simulink model "car_model_FIXED"  (R2022b)
settings: Solver=VariableStepAuto  StartTime=0.0  StopTime=60  RelTol=1e-3
values from neighbouring files (symbols this model uses):
  ABS_MAX_TORQUE = [25 25 25 25]    [Startup.m]
  ABS_MAX_TRQ_CMD = dot(ABS_MAX_TORQUE, MOTOR_ENABLE)    [Startup.m]
  ABS_MIN_TORQUE = [0.01 0.01 0.01 0.01]    [Startup.m]
  acc_IC = 0    [Startup.m]
  ACCELERATION_MAX = 30    [Startup.m]
  ang_IC = 0    [Startup.m]
  ang_vel_IC = 0    [Startup.m]
  ax = Reference_Signals.Chassis_Acceleration_VNED.ax.Data(:)    [Simulation_Data_Parse.m]    (also in Vehicle_Sim_Parse.m)
  ay = Reference_Signals.Chassis_Acceleration_VNED.ay.Data(:)    [Simulation_Data_Parse.m]    (also in Vehicle_Sim_Parse.m)
  az = Reference_Signals.Chassis_Acceleration_VNED.az.Data(:)    [Simulation_Data_Parse.m]    (also in Vehicle_Sim_Parse.m)
  battery_current_IC = 0    [Startup.m]
  BATTERY_CURRENT_MAX = 140    [Startup.m]
  BATTERY_CURRENT_MIN = 0    [Startup.m]
  battery_FT_IC = 300    [Startup.m]
  battery_T_IC = 300    [Startup.m]
  BATTERY_TEMPERATURE_MAX = 60    [Startup.m]
  BATTERY_TEMPERATURE_MIN = 0    [Startup.m]
  battery_voltage_IC = Ns*max(Em)    [Startup.m]
  BATTERY_VOLTAGE_MAX = 340    [Startup.m]
  BATTERY_VOLTAGE_MIN = 60    [Startup.m]
  Brake_Pressure_IC = 1    [Startup.m]
  ccl_IC = 0    [Startup.m]
  CENTER_STEER_ANGLE_MAX = 130    [Startup.m]
  covarience_matrix_IC = Simulink.Parameter(eye(28)./1000)    [Startup.m]
  dcl_IC = 140    [Startup.m]
  DCL_MAX = 130    [Startup.m]
  DCL_MIN = 0    [Startup.m]
  driver_t = 0.015    [Startup.m]
  fusion_t = Simulink.Parameter(0.01)    [Startup.m]
  fusion_t_sim = fusion_t.copy    [Startup.m]
  Fz_IC = m_all*g/4    [Startup.m]
  g = 9.81    [Startup.m]
  gps_hz = 0.01    [Startup.m]
  gps_ratio = Simulink.Parameter(gps_hz / imu_hz.Value)    [Startup.m]
  imu_hz = fusion_t.copy    [Startup.m]
  location_lla_IC = Simulink.Parameter([40.437675, -86.943750, 200])    [Startup.m]
  MAG_MAX = 200    [Startup.m]
  Max_Brake_Pressure = 10^8    (= 100000000)    [Startup.m]
  Max_Driver_Input = 1    [Startup.m]
  MAX_DTHETA_DRIVER = 360    [Startup.m]
  MAX_STEERING_ADJUST = 15    [Startup.m]
  Min_Brake_Pressure = 1    [Startup.m]
  Min_Driver_Input = 0    [Startup.m]
  motor_current_IC = 0    [Startup.m]
  MOTOR_CURRENT_MAX = 70    [Startup.m]
  MOTOR_CURRENT_MIN = 0    [Startup.m]
  MOTOR_ENABLE = [0 0 1 1]    [Startup.m]
  motor_FT_IC = 300    [Startup.m]
  motor_T_IC = 300    [Startup.m]
  MOTOR_TEMPERATURE_MAX = 100    [Startup.m]
  MOTOR_TEMPERATURE_MIN = 0    [Startup.m]
  motor_voltage_IC = 332    [Startup.m]
  MOTOR_VOLTAGE_MAX = 340    [Startup.m]
  MOTOR_VOLTAGE_MIN = 90    [Startup.m]
  omega_IC = 0    [Startup.m]
  OMEGA_MAX = 150    [Startup.m]
  OMEGA_MIN = 0    [Startup.m]
  ORIENTATION_MAX = 360    [Startup.m]
  pos_IC = 0    [Startup.m]
  POS_MAX = 300    [Startup.m]
  rho = 1.225    [Startup.m]
  selected_maxvm = MIN_TRACK_DATA.(event_names(10))    [Startup.m]
  selected_sweep = ALL_SWEEP_DATA.(sweep_names(1))    [Startup.m]
  selected_track = ALL_TRACK_DATA.(event_names(10))    [Startup.m]
  shock_length_IC = 0.1    [Startup.m]
  SHOCK_LENGTH_MAX = 0.25    [Startup.m]
  SHOCK_LENGTH_MIN = 0    [Startup.m]
  state_IC = zeros(28,1)    [Startup.m]
  theta_IC = 0    [Startup.m]
  TRACTION_ENABLE = 0    [Startup.m]
  TVS_ENABLE = 0    [Startup.m]
  tvs_t = 0.015    [Startup.m]
  tvs_t_sim = tvs_t    (= 0.015)    [Startup.m]
  Tx_I = 0    [Startup.m]
  vel_IC = [0 0 0]    [Startup.m]
  VELOCITY_MAX = 30    [Startup.m]
  X = Reference_Signals.Chassis_Position.X.Data(:)    [Simulation_Data_Parse.m]    (also in Vehicle_Sim_Parse.m = Chassis_Signals.InertFrm.Cg.Disp.X.Data(:))
  Y = Reference_Signals.Chassis_Position.Y.Data(:)    [Simulation_Data_Parse.m]    (also in Vehicle_Sim_Parse.m = Chassis_Signals.InertFrm.Cg.Disp.Y.Data(:))
  YAW_ENABLE = 1    [Startup.m]
  YAW_MAX = 2.5    [Startup.m]
undefined symbols (not defined in the file or in its folder): ActSuspDutyCycle, Aeq_left, Aeq_right, alpha_error, ang_acc_hystersesis, area_air, axb, br, brake_bias, covA, covG, covM, covP, covV, CURRENT_BUFFER, cy_sweep, dB, deadband_angle, dIndex, DiscIntNeverNeededParam, dt_OFF, dt_ON, dTx, dx, dZ, efficiency_grid, F0z, forward_look_straight, forward_look_turn, Fz_sweep, GAIN_ABS, gearbox_efficiency, gr, I, I_Driver, IMU_accel, IMU_gyro, IMU_mag, IMUNED2VNED, indicies, IYY, kx_sweep, l, lambda_star, low_V_SA, lr, m_all, m_body, m_unsprung, MAGNED2VNED, MAX_I_Driver, max_yaw, min_velocity_regen, motorControllerCurve, motorTempCurve, motorTempX, mu_star, mx_sweep, my_sweep, noise_state ... (+40)
libraries: fl_lib x82, nesl_utility x32, vehdynlibtire x10, vehdynlibsuspension x8, simulink x5, autolibutils x5, sharedtransform x5, sdl_lib x4, EngineCoolingComponents_lib x4, slpidlib x3, SimscapeFluids_lib x3, shared6dof x2
(part 2 of 14)

== system car_model_FIXED/Driver & Environment/Reference Generator ==
  Analog Signals : Inport
  Driver Information : BusCreator  Inputs=12
  Memory : Memory  InitialCondition=1
  Memory1 : Memory  InitialCondition=1
  Reference Geneator : MATLAB Function  TreatAsAtomicUnit=on  SystemSampleTime=driver_t
  Selector : BusSelector  OutputSignals=psi,Vel,r,Disp,Omega
  Subsystem : Subsystem
  To Workspace : ToWorkspace  VariableName=Driver_Signals  SaveFormat=Timeseries  SampleTime=-1
  Unit Delay : UnitDelay  SampleTime=-1  HasFrameUpgradeWarning=on
  Unit Delay1 : UnitDelay  InitialCondition=1000  SampleTime=-1  HasFrameUpgradeWarning=on
  Controller Information : Outport
  wires:
  Analog Signals/1 -> To Workspace/1, Selector/1  "Driver"
  Selector/1 -> Subsystem/1(<psi>)  "<psi>"
  Reference Geneator/4(d_error) -> Driver Information/2
  Driver Information/1 -> Controller Information/1  "Driver Information"
  Selector/2 -> Reference Geneator/4(Vg)  "<Vel>"
  Reference Geneator/3(v_error) -> Driver Information/1
  Reference Geneator/6(v_cog) -> Driver Information/4
  Subsystem/1(psi_rev) -> Reference Geneator/3(psi)
  Reference Geneator/5(psi_error) -> Driver Information/3
  Reference Geneator/2(index_all) -> Memory/1
  Memory/1 -> Reference Geneator/2("index_all ")
  Reference Geneator/7(r_ref) -> Driver Information/5
  Reference Geneator/8(r_error) -> Driver Information/6
  Reference Geneator/15(ahead) -> Unit Delay/1
  Unit Delay/1 -> Reference Geneator/8("ahead ")
  Reference Geneator/12(omega) -> Driver Information/10
  Reference Geneator/9(x_ref) -> Driver Information/7
  Reference Geneator/10(y_ref) -> Driver Information/8
  Selector/3 -> Reference Geneator/5(yaw)  "<r>"
  Selector/4 -> Reference Geneator/6(pos)  "<Disp>"
  Reference Geneator/11(yaw_ref) -> Driver Information/9
  Memory1/1 -> Reference Geneator/1("index_small ")
  Reference Geneator/1(index_small) -> Memory1/1
  Reference Geneator/16(di_now) -> Unit Delay1/1
  Unit Delay1/1 -> Reference Geneator/9(di_prev)
  Selector/5 -> Reference Geneator/7("omega ")  "<Omega>"
  Reference Geneator/13(p_error) -> Driver Information/11
  Reference Geneator/14(Vnow) -> Driver Information/12

== system car_model_FIXED/Driver & Environment/Sweep Generator ==
  Analog Signals : Inport
  Bus Creator : BusCreator  Inputs=2
  Bus Selector : BusSelector  OutputSignals=Vel
  Memory : Memory  InitialCondition=1
  Sweep Generator : MATLAB Function  TreatAsAtomicUnit=on  SystemSampleTime=driver_t
  To Workspace : ToWorkspace  VariableName=counter  SaveFormat=Timeseries  SampleTime=-1
  Unit Delay : UnitDelay  SampleTime=-1  HasFrameUpgradeWarning=on
  Unit Delay1 : UnitDelay  InitialCondition=1  SampleTime=-1  HasFrameUpgradeWarning=on
  Controller Information : Outport
  wires:
  Analog Signals/1 -> Bus Selector/1
  Sweep Generator/2(vel_err) -> Bus Creator/1  "Velocity Error"
  Sweep Generator/3(ref_steer) -> Bus Creator/2  "Steering Angle"
  Bus Creator/1 -> Controller Information/1
  Bus Selector/1 -> Sweep Generator/2(vel)  "<Vel>"
  Sweep Generator/1(index) -> Memory/1
  Memory/1 -> Sweep Generator/1("index ")
  Sweep Generator/5(counter) -> Unit Delay/1, To Workspace/1
  Unit Delay/1 -> Sweep Generator/4("counter ")
  Sweep Generator/4(ON) -> Unit Delay1/1
  Unit Delay1/1 -> Sweep Generator/3("ON ")

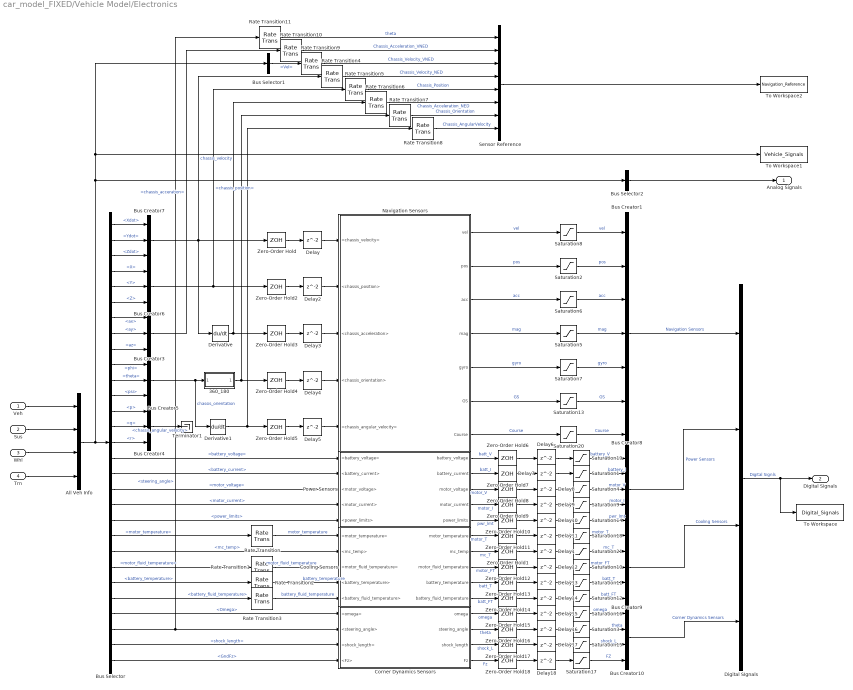
== system car_model_FIXED/Vehicle Model/Electronics ==
  Veh : Inport
  Sus : Inport  Port=2
  Whl : Inport  Port=3
  Trn : Inport  Port=4
  360_180 : Subsystem
  All Veh Info : BusCreator  Inputs=veh,sus,whl,trn
  Bus Creator1 : BusCreator  Inputs=7
  Bus Creator10 : BusCreator  Inputs=4
  Bus Creator3 : BusCreator  Inputs=ax,ay,az
  Bus Creator4 : BusCreator  Inputs=p,q,r
  Bus Creator5 : BusCreator  Inputs=phi,theta,psi
  Bus Creator6 : BusCreator  Inputs=X,Y,Z
  Bus Creator7 : BusCreator  Inputs=Xdot,Ydot,Zdot
  Bus Creator8 : BusCreator  Inputs=5
  Bus Creator9 : BusCreator  Inputs=5
  Bus Selector : BusSelector  OutputSignals=veh.InertFrm.Cg.Vel.Xdot,veh.InertFrm.Cg.Vel.Ydot,veh.InertFrm.Cg.Vel.Zdot,veh.InertFrm.Cg.Disp.X,veh.InertFrm.Cg.Disp.Y,veh.InertFrm.Cg.Disp.Z,veh.BdyFrm.Cg.Acc.ax,veh.BdyFrm.Cg.Acc.ay,veh.BdyFrm.Cg.Acc.az,veh.InertFrm.Cg.Ang.phi,veh.InertFrm.Cg.Ang.theta,veh.InertFrm.Cg.Ang.psi,veh.BdyFrm.Cg.AngVel.p,veh.BdyFrm.Cg.AngVel.q,veh.BdyFrm.Cg.AngVel.r,trn.battery_voltage,trn.battery_current,trn.motor_voltage,trn.motor_current,trn.power_limits,trn.motor_temperature,trn.mc_temp,trn.motor_fluid_temperature,trn.battery_temperature,trn.battery_fluid_temperature,whl.TireFrame.Omega,sus.Sus.steering_angle,sus.Sus.shock_length,whl.TireFrame.GndFz
  Bus Selector1 : BusSelector  OutputSignals=veh.BdyFrm.Cg.Vel
  Bus Selector2 : BusSelector  OutputSignals=veh.InertFrm.Cg.Disp,veh.InertFrm.Cg.Ang.psi,veh.BdyFrm.Cg.Vel,veh.BdyFrm.Cg.AngVel.r,sus.Sus.steering_angle,whl.TireFrame.Omega  OutputAsBus=on
  Cooling Sensors : Subsystem
  Corner Dynamics Sensors : Subsystem
  Delay : Delay  InitialCondition=([1;1]*vel_IC)'
  Delay1 : Delay  InitialCondition=[1 1; 1 1; 1 1; 1 1].*motor_T_IC
  Delay10 : Delay  InitialCondition=[dcl_IC; ccl_IC]*[1 1]
  Delay11 : Delay  InitialCondition=[1 1; 1 1; 1 1; 1 1].*motor_T_IC
  Delay12 : Delay  InitialCondition=[1 1; 1 1].*motor_FT_IC
  Delay13 : Delay  InitialCondition=[1 1].*battery_T_IC
  Delay14 : Delay  InitialCondition=[1 1].*battery_FT_IC
  Delay15 : Delay  InitialCondition=ones(1, 4, 2).*omega_IC
  Delay16 : Delay  InitialCondition=[1 1].*theta_IC
  Delay17 : Delay  InitialCondition=[1 1; 1 1; 1 1; 1 1].*shock_length_IC
  Delay18 : Delay  InitialCondition=[1 1; 1 1; 1 1; 1 1].*Fz_IC
  Delay2 : Delay  InitialCondition=[1 1; 1 1; 1 1].*pos_IC
  Delay3 : Delay  InitialCondition=[1 1; 1 1; 1 1].*acc_IC
  Delay4 : Delay  InitialCondition=[1 1; 1 1; 1 1].*ang_IC
  Delay5 : Delay  InitialCondition=[1 1; 1 1; 1 1].*ang_vel_IC
  Delay6 : Delay  InitialCondition=[1 1].*battery_voltage_IC
  Delay7 : Delay  InitialCondition=[1 1].*battery_current_IC
  Delay8 : Delay  InitialCondition=[1 1; 1 1; 1 1; 1 1].*motor_voltage_IC
  Delay9 : Delay  InitialCondition=ones(1, 4, 2).*motor_current_IC
  Derivative : Derivative
  Derivative1 : Derivative
  Digital SIgnals : BusCreator  Inputs=4
  Navigation Sensors : Subsystem
  Power Sensors : Subsystem
  Rate Transition : RateTransition  OutPortSampleTime=0
  Rate Transition1 : RateTransition  InitialCondition=[1 1].*motor_FT_IC  OutPortSampleTime=0
  Rate Transition{4..11} (8 alike) : RateTransition  Deterministic=off  OutPortSampleTime=fusion_t
  Rate Transition2 : RateTransition  OutPortSampleTime=0
  Rate Transition3 : RateTransition  OutPortSampleTime=0
  Saturation1 : Saturate  UpperLimit=BATTERY_CURRENT_MAX  LowerLimit=BATTERY_CURRENT_MIN
  Saturation10 : Saturate  UpperLimit=MOTOR_TEMPERATURE_MAX  LowerLimit=MOTOR_TEMPERATURE_MIN
  Saturation11 : Saturate  UpperLimit=BATTERY_TEMPERATURE_MAX  LowerLimit=BATTERY_TEMPERATURE_MIN
  Saturation12 : Saturate  UpperLimit=BATTERY_TEMPERATURE_MAX  LowerLimit=BATTERY_TEMPERATURE_MIN
  Saturation13 : Saturate  UpperLimit=VELOCITY_MAX  LowerLimit=-VELOCITY_MAX
  Saturation14 : Saturate  UpperLimit=DCL_MAX  LowerLimit=DCL_MIN
  Saturation15 : Saturate  UpperLimit=SHOCK_LENGTH_MAX  LowerLimit=SHOCK_LENGTH_MIN
  Saturation16 : Saturate  UpperLimit=OMEGA_MAX  LowerLimit=OMEGA_MIN
  Saturation17 : Saturate  UpperLimit=1200  LowerLimit=200
  Saturation18 : Saturate  UpperLimit=MOTOR_TEMPERATURE_MAX  LowerLimit=MOTOR_TEMPERATURE_MIN
  Saturation19 : Saturate  UpperLimit=BATTERY_VOLTAGE_MAX  LowerLimit=BATTERY_VOLTAGE_MIN
  Saturation2 : Saturate  UpperLimit=inf  LowerLimit=-inf
  Saturation20 : Saturate  UpperLimit=ORIENTATION_MAX  LowerLimit=-ORIENTATION_MAX
  Saturation21 : Saturate  UpperLimit=MOTOR_TEMPERATURE_MAX  LowerLimit=MOTOR_TEMPERATURE_MIN
  Saturation3 : Saturate  UpperLimit=CENTER_STEER_ANGLE_MAX  LowerLimit=-CENTER_STEER_ANGLE_MAX
  Saturation4 : Saturate  UpperLimit=MOTOR_VOLTAGE_MAX  LowerLimit=MOTOR_VOLTAGE_MIN
  Saturation5 : Saturate  UpperLimit=MAG_MAX  LowerLimit=-MAG_MAX
  Saturation6 : Saturate  UpperLimit=ACCELERATION_MAX  LowerLimit=-ACCELERATION_MAX
  Saturation7 : Saturate  UpperLimit=YAW_MAX  LowerLimit=-YAW_MAX
  Saturation8 : Saturate  UpperLimit=VELOCITY_MAX  LowerLimit=-VELOCITY_MAX
  Saturation9 : Saturate  UpperLimit=MOTOR_CURRENT_MAX  LowerLimit=MOTOR_CURRENT_MIN
  Sensor Reference : BusCreator  Inputs=8
  Terminator1 : Terminator
  To Workspace : ToWorkspace  VariableName=Digital_Signals  SaveFormat=Timeseries  SampleTime=-1
  To Workspace1 : ToWorkspace  VariableName=Vehicle_Signals  SaveFormat=Timeseries  SampleTime=-1
  To Workspace2 : ToWorkspace  VariableName=Navigation_Reference  SaveFormat=Timeseries  SampleTime=-1
  Zero-Order Hold : ZeroOrderHold  SampleTime=gps_hz
  Zero-Order Hold{1,6..18} (14 alike) : ZeroOrderHold  SampleTime=tvs_t_sim
  Zero-Order Hold2 : ZeroOrderHold  SampleTime=gps_hz
  Zero-Order Hold3 : ZeroOrderHold  SampleTime=imu_hz
  Zero-Order Hold4 : ZeroOrderHold  SampleTime=imu_hz
  Zero-Order Hold5 : ZeroOrderHold  SampleTime=imu_hz
  Analog Signals : Outport
  Digital Signals : Outport  Port=2
  wires:
  Sus/1 -> All Veh Info/2
  Whl/1 -> All Veh Info/3
  Veh/1 -> All Veh Info/1
  Trn/1 -> All Veh Info/4
  Bus Selector/7 -> Bus Creator3/1  "<ax>"
  Bus Selector/8 -> Bus Creator3/2  "<ay>"
  Bus Selector/9 -> Bus Creator3/3  "<az>"
  Bus Selector/13 -> Bus Creator4/1  "<p>"
  Bus Selector/14 -> Bus Creator4/2  "<q>"
  Bus Selector/15 -> Bus Creator4/3  "<r>"
  Bus Selector/1 -> Bus Creator7/1  "<Xdot>"
  Bus Selector/2 -> Bus Creator7/2  "<Ydot>"
  Bus Selector/10 -> Bus Creator5/1  "<phi>"
  Bus Selector/11 -> Bus Creator5/2  "<theta>"
  Bus Selector/12 -> Bus Creator5/3  "<psi>"
  Bus Selector/4 -> Bus Creator6/1  "<X>"
  Bus Selector/5 -> Bus Creator6/2  "<Y>"
  Bus Selector2/1 -> Analog Signals/1
  Bus Selector/3 -> Bus Creator7/3  "<Zdot>"
  Bus Selector/6 -> Bus Creator6/3  "<Z>"
  Bus Creator7/1 -> Zero-Order Hold/1, Rate Transition4/1, Derivative/1  "chassis_velocity"
  Bus Creator6/1 -> Zero-Order Hold2/1, Rate Transition5/1  "<chassis_position>"
  Bus Creator5/1 -> Derivative1/1, 360_180/1(<psi>)  "chassis_orientation"
  Bus Selector/20 -> Power Sensors/5(<power_limits>)  "<power_limits>"
  Bus Selector/17 -> Power Sensors/2(<battery_current>)  "<battery_current>"
  Bus Selector/19 -> Power Sensors/4(<motor_current>)  "<motor_current>"
  Bus Selector/18 -> Power Sensors/3(<motor_voltage>)  "<motor_voltage>"
  Bus Selector/21 -> Rate Transition/1  "<motor_temperature>"
  Bus Selector/26 -> Corner Dynamics Sensors/1(<omega>)  "<Omega>"
  Bus Selector/27 -> Corner Dynamics Sensors/2(<steering_angle>), Rate Transition11/1  "<steering_angle>"
  Bus Selector/28 -> Corner Dynamics Sensors/3(<shock_length>)  "<shock_length>"
  Bus Selector/29 -> Corner Dynamics Sensors/4(<Fz>)  "<GndFz>"
  Bus Selector/23 -> Rate Transition1/1  "<motor_fluid_temperature>"
  Bus Selector/16 -> Power Sensors/1(<battery_voltage>)  "<battery_voltage>"
  Bus Selector/24 -> Rate Transition2/1  "<battery_temperature>"
  Bus Selector/25 -> Rate Transition3/1  "<battery_fluid_temperature>"
  Navigation Sensors/1(vel) -> Saturation8/1  "vel"
  Navigation Sensors/2(pos) -> Saturation2/1  "pos"
  Navigation Sensors/3(acc) -> Saturation6/1  "acc"
  Navigation Sensors/4(mag) -> Saturation5/1  "mag"
  Navigation Sensors/5(gyro) -> Saturation7/1  "gyro"
  Power Sensors/1(battery_voltage) -> Zero-Order Hold6/1  "batt_V"
  Power Sensors/2(battery_current) -> Zero-Order Hold7/1  "batt_I"
  Power Sensors/3(motor_voltage) -> Zero-Order Hold8/1  "motor_V"
  Power Sensors/4(motor_current) -> Zero-Order Hold9/1  "motor_I"
  Power Sensors/5(power_limits) -> Zero-Order Hold10/1  "pwr_lmt"
  Cooling Sensors/1(motor_temperature) -> Zero-Order Hold11/1  "motor_T"
  Cooling Sensors/3(motor_fluid_temperature) -> Zero-Order Hold12/1  "motor_FT"
  Cooling Sensors/4(battery_temperature) -> Zero-Order Hold13/1  "batt_T"
  Cooling Sensors/5(battery_fluid_temperature) -> Zero-Order Hold14/1  "batt_FT"
  Corner Dynamics Sensors/1(omega) -> Zero-Order Hold15/1  "omega"
  Corner Dynamics Sensors/2(steering_angle) -> Zero-Order Hold16/1  "theta"
  Corner Dynamics Sensors/3(shock_length) -> Zero-Order Hold17/1  "shock_L"
  Corner Dynamics Sensors/4(Fz) -> Zero-Order Hold18/1  "Fz"
  Bus Creator1/1 -> Digital SIgnals/1  "Navigation Sensors"
  Bus Creator8/1 -> Digital SIgnals/2  "Power Sensors"
  Bus Creator10/1 -> Digital SIgnals/4  "Corner Dynamics Sensors"
  Digital SIgnals/1 -> Digital Signals/1, To Workspace/1  "Digital Signls"
  Saturation15/1 -> Bus Creator10/3  "shock_L"
  Saturation17/1 -> Bus Creator10/4  "FZ"
  Saturation3/1 -> Bus Creator10/2  "theta"
  Saturation16/1 -> Bus Creator10/1  "omega"
  Saturation8/1 -> Bus Creator1/1  "vel"
  Saturation2/1 -> Bus Creator1/2  "pos"
  Saturation6/1 -> Bus Creator1/3  "acc"
  Saturation5/1 -> Bus Creator1/4  "mag"
  Saturation7/1 -> Bus Creator1/5  "gyro"
  Saturation19/1 -> Bus Creator8/1  "battery_V"
  Saturation1/1 -> Bus Creator8/2  "battery_I"
  Saturation9/1 -> Bus Creator8/4  "motor_I"
  Saturation4/1 -> Bus Creator8/3  "motor_V"
  Saturation14/1 -> Bus Creator8/5  "pwr_lmt"
  Saturation18/1 -> Bus Creator9/1  "motor_T"
  Saturation10/1 -> Bus Creator9/3  "motor_FT"
  Saturation11/1 -> Bus Creator9/4  "batt_T"
  Saturation12/1 -> Bus Creator9/5  "batt_FT"
  Zero-Order Hold6/1 -> Delay6/1
  Zero-Order Hold7/1 -> Delay7/1
  Zero-Order Hold8/1 -> Delay8/1
  Zero-Order Hold9/1 -> Delay9/1
  Zero-Order Hold10/1 -> Delay10/1
  Zero-Order Hold11/1 -> Delay11/1
  Zero-Order Hold12/1 -> Delay12/1
  Zero-Order Hold13/1 -> Delay13/1
  Zero-Order Hold14/1 -> Delay14/1
  Zero-Order Hold15/1 -> Delay15/1
  Zero-Order Hold16/1 -> Delay16/1
  Zero-Order Hold17/1 -> Delay17/1
  Zero-Order Hold18/1 -> Delay18/1
  Delay6/1 -> Saturation19/1
  Delay7/1 -> Saturation1/1
  Delay8/1 -> Saturation4/1
  Delay9/1 -> Saturation9/1
  Delay10/1 -> Saturation14/1
  Delay11/1 -> Saturation18/1
  Delay12/1 -> Saturation10/1
  Delay13/1 -> Saturation11/1
  Delay14/1 -> Saturation12/1
  Delay15/1 -> Saturation16/1
  Delay16/1 -> Saturation3/1
  Delay17/1 -> Saturation15/1
  Delay18/1 -> Saturation17/1
  Rate Transition/1 -> Cooling Sensors/1(<motor_temperature>)  "motor_temperature"
  Rate Transition1/1 -> Cooling Sensors/3(<motor_fluid_temperature>)  "motor_fluid_temperature"
  Rate Transition2/1 -> Cooling Sensors/4(<battery_temperature>)  "battery_temperature"
  Rate Transition3/1 -> Cooling Sensors/5(<battery_fluid_temperature>)  "battery_fluid_temperature"
  Bus Creator9/1 -> Digital SIgnals/3  "Cooling Sensors"
  Navigation Sensors/6(GS) -> Saturation13/1  "GS"
  Navigation Sensors/7(Course) -> Saturation20/1  "Course"
  Saturation13/1 -> Bus Creator1/6  "GS"
  Saturation20/1 -> Bus Creator1/7  "Course"
  Delay/1 -> Navigation Sensors/1(<chassis_velocity>)
  Delay2/1 -> Navigation Sensors/2(<chassis_position>)
  Derivative/1 -> Zero-Order Hold3/1, Rate Transition6/1
  360_180/1(psi_rev) -> Zero-Order Hold4/1, Rate Transition7/1
  Delay3/1 -> Navigation Sensors/3(<chassis_acceleration>)
  Delay4/1 -> Navigation Sensors/4(<chassis_orientation>)
  Delay5/1 -> Navigation Sensors/5(<chassis_angular_velocity>)
  Derivative1/1 -> Zero-Order Hold5/1, Rate Transition8/1
  Sensor Reference/1 -> To Workspace2/1
  Rate Transition4/1 -> Sensor Reference/4  "Chassis_Velocity_NED"
  Rate Transition5/1 -> Sensor Reference/5  "Chassis_Position"
  Rate Transition6/1 -> Sensor Reference/6  "Chassis_Acceleration_NED"
  Rate Transition7/1 -> Sensor Reference/7  "Chassis_Orientation"
  Rate Transition8/1 -> Sensor Reference/8  "Chassis_AngularVelocity"
  Bus Creator4/1 -> Terminator1/1  "<chassis_angular_velocity>"
  Bus Creator3/1 -> Rate Transition10/1  "<chassis_acceration>"
  Zero-Order Hold/1 -> Delay/1
  Zero-Order Hold2/1 -> Delay2/1
  Zero-Order Hold3/1 -> Delay3/1
  Zero-Order Hold4/1 -> Delay4/1
  Zero-Order Hold5/1 -> Delay5/1
  Bus Selector/22 -> Cooling Sensors/2(<mc_temp>)  "<mc_temp>"
  Zero-Order Hold1/1 -> Delay1/1
  Delay1/1 -> Saturation21/1
  Cooling Sensors/2(mc_temp) -> Zero-Order Hold1/1  "mc_T"
  Saturation21/1 -> Bus Creator9/2  "mc_T"
  All Veh Info/1 -> Bus Selector1/1, To Workspace1/1, Bus Selector2/1, Bus Selector/1
  Bus Selector1/1 -> Rate Transition9/1  "<Vel>"
  Rate Transition9/1 -> Sensor Reference/3  "Chassis_Velocity_VNED"
  Rate Transition10/1 -> Sensor Reference/2  "Chassis_Acceleration_VNED"
  Rate Transition11/1 -> Sensor Reference/1  "theta"
